simulink model "UrbanCHIL"  (Simulink 8.1)
settings: Solver=ode1  StartTime=0.0  StopTime=inf  FixedStep=Ts  MaxStep=1e-3  RelTol=1e-3
PostLoadFcn:
  | NREL_Mode=1; BANSHEE_init;
InitFcn:
  | NREL_Mode=1; BANSHEE_init;
values from neighbouring files (symbols this model uses):
  DER_REL = xlsread('DER_relay.xlsx')    [relay_settings_init.m]
  F0 = xlsread('F0_relay_banshee.xlsx')    [relay_settings_init.m]
  F2 = xlsread('F2_relay_banshee.xlsx')    [relay_settings_init.m]
  F3 = xlsread('F3_relay_banshee.xlsx')    [relay_settings_init.m]
  F4 = xlsread('F4_relay_nrel.xlsx')    [relay_settings_init.m]
  Ts = 100E-6    (= 0.0001)    [BANSHEE_init.m]    (also in Ghost_init.m)
undefined symbols (not defined in the file or in its folder): CBID, communications_lib, Feeder2_lib, Feeder3_lib, Feeder4_lib, generic_ethernet_cb, Left, relay_housing_lib, SM_UtilityService, SS_COMMUNICATION, SS_F2_RELAY_HOUSING, SS_F3_RELAY_HOUSING, SS_Feeder2, SS_Feeder3, SS_Feeder4, Stim, type, utility_service_lib, V
libraries: simulink x80, relay_modbus_lib x80, breaker_lib x46, rtio_generic_modbus x45, cables_lib x30, rtlab x22, Load_lib x21, powerlib x20, transformer_lib x19, ssn_lib x13, artemis x6, BESS_lib x4
(part 6 of 6)

== system UrbanCHIL/SS_COMMUNICATION/Relay_data/ExtractF3 ==
  In1 : Inport
  Bus Selector47 : BusSelector  OutputSignals=F3_CB_1,F3_CB_2,F3_CB_3,F3_CB_4,F3_CB_5,F3_CB_6,F3_CB_7,F3_CB_8,F3_CB_9,F3_CB_10
  Bus Selector{48..53,56,58..59,61} (10 alike) : BusSelector  OutputSignals=m.kw,m.kvar,m.Vpu,m.Hz,m.status  OutputAsBus=on
  Mux13 : Mux  Inputs=10
  Out1 : Outport
  wires:
  Bus Selector51/1 -> Mux13/5
  Bus Selector48/1 -> Mux13/1
  Bus Selector53/1 -> Mux13/7
  Bus Selector47/4 -> Bus Selector50/1  "<F3_CB_4>"
  Bus Selector47/1 -> Bus Selector48/1  "<F3_CB_1>"
  Bus Selector50/1 -> Mux13/4
  In1/1 -> Bus Selector47/1
  Mux13/1 -> Out1/1
  Bus Selector52/1 -> Mux13/6
  Bus Selector56/1 -> Mux13/8
  Bus Selector58/1 -> Mux13/9
  Bus Selector47/6 -> Bus Selector52/1  "<F3_CB_6>"
  Bus Selector47/7 -> Bus Selector53/1  "<F3_CB_7>"
  Bus Selector47/8 -> Bus Selector56/1  "<F3_CB_8>"
  Bus Selector47/9 -> Bus Selector58/1  "<F3_CB_9>"
  Bus Selector47/3 -> Bus Selector61/1  "<F3_CB_3>"
  Bus Selector47/2 -> Bus Selector49/1  "<F3_CB_2>"
  Bus Selector49/1 -> Mux13/2
  Bus Selector47/10 -> Bus Selector59/1  "<F3_CB_10>"
  Bus Selector47/5 -> Bus Selector51/1  "<F3_CB_5>"
  Bus Selector59/1 -> Mux13/10
  Bus Selector61/1 -> Mux13/3

== system UrbanCHIL/SS_COMMUNICATION/Relay_data/ExtractF4 ==
  In1 : Inport
  Bus Selector47 : BusSelector  OutputSignals=F4_CB_1,F4_CB_2,F4_CB_3,F4_CB_4,F4_CB_5,F4_CB_6
  Bus Selector{48..52,61} (6 alike) : BusSelector  OutputSignals=m.kw,m.kvar,m.Vpu,m.Hz,m.status  OutputAsBus=on
  Mux13 : Mux  Inputs=6
  Out1 : Outport
  wires:
  Bus Selector61/1 -> Mux13/3
  Bus Selector47/5 -> Bus Selector51/1  "<F4_CB_5>"
  Bus Selector49/1 -> Mux13/2
  Bus Selector47/2 -> Bus Selector49/1  "<F4_CB_2>"
  Bus Selector47/3 -> Bus Selector61/1  "<F4_CB_3>"
  Bus Selector47/6 -> Bus Selector52/1  "<F4_CB_6>"
  Bus Selector52/1 -> Mux13/6
  Mux13/1 -> Out1/1
  In1/1 -> Bus Selector47/1
  Bus Selector50/1 -> Mux13/4
  Bus Selector47/1 -> Bus Selector48/1  "<F4_CB_1>"
  Bus Selector47/4 -> Bus Selector50/1  "<F4_CB_4>"
  Bus Selector48/1 -> Mux13/1
  Bus Selector51/1 -> Mux13/5

== system UrbanCHIL/SS_COMMUNICATION/Relay_data/Subsystem ==
  F2 : Inport
  F3 : Inport  Port=2
  Bus Selector1 : BusSelector  OutputSignals=F2_PCC
  Bus Selector2 : BusSelector  OutputSignals=m.kw,m.kvar,m.Vpu,m.Hz,m.status  OutputAsBus=on
  Bus Selector3 : BusSelector  OutputSignals=F3_PCC
  Bus Selector4 : BusSelector  OutputSignals=m.kw,m.kvar,m.Vpu,m.Hz,m.status  OutputAsBus=on
  Constant3 : Constant  Value=zeros(1,5)
  Mux : Mux  Inputs=3
  Out1 : Outport
  wires:
  Constant3/1 -> Mux/1
  Bus Selector1/1 -> Bus Selector2/1  "<F2_PCC>"
  F2/1 -> Bus Selector1/1
  Bus Selector2/1 -> Mux/2
  Bus Selector3/1 -> Bus Selector4/1  "<F3_PCC>"
  F3/1 -> Bus Selector3/1
  Bus Selector4/1 -> Mux/3
  Mux/1 -> Out1/1

== system UrbanCHIL/SS_COMMUNICATION/Relay_data/Subsystem1 ==
  F2 : Inport
  F3 : Inport  Port=2
  F4 : Inport  Port=3
  Bus Selector1 : BusSelector  OutputSignals=ESS_DATA,PV_DATA
  Bus Selector10 : BusSelector  OutputSignals=m.kw,m.kvar,m.Vpu,m.Hz,m.status  OutputAsBus=on
  Bus Selector11 : BusSelector  OutputSignals=cb.relay_out
  Bus Selector{2,6,12,17} (4 alike) : BusSelector  OutputSignals=CB_meas.relay_out.m.kw,CB_meas.relay_out.m.kvar,CB_meas.relay_out.m.Vpu,CB_meas.relay_out.m.Hz,CB_meas.cb_meas.Status  OutputAsBus=on
  Bus Selector16 : BusSelector  OutputSignals=cb.relay_out
  Bus Selector3 : BusSelector  OutputSignals=NG_CHP_DATA
  Bus Selector4 : BusSelector  OutputSignals=m.kw,m.kvar,m.Vpu,m.Hz,m.status  OutputAsBus=on
  Bus Selector9 : BusSelector  OutputSignals=GEN3_DATA,ESS_DATA,PV_DATA
  Constant3 : Constant  Value=zeros(1,5)
  Mux : Mux  Inputs=7
  Out1 : Outport
  wires:
  Mux/1 -> Out1/1
  Bus Selector4/1 -> Mux/4
  F3/1 -> Bus Selector3/1
  Bus Selector3/1 -> Bus Selector16/1  "<NG_CHP_DATA>"
  Bus Selector6/1 -> Mux/2
  F2/1 -> Bus Selector1/1
  Bus Selector1/1 -> Bus Selector6/1  "<ESS_DATA>"
  Constant3/1 -> Mux/1
  Bus Selector1/2 -> Bus Selector2/1  "<PV_DATA>"
  Bus Selector2/1 -> Mux/3
  F4/1 -> Bus Selector9/1
  Bus Selector9/1 -> Bus Selector11/1  "<GEN3_DATA>"
  Bus Selector11/1 -> Bus Selector10/1  "<relay_out>"
  Bus Selector10/1 -> Mux/5
  Bus Selector17/1 -> Mux/6
  Bus Selector9/3 -> Bus Selector12/1  "<PV_DATA>"
  Bus Selector12/1 -> Mux/7
  Bus Selector16/1 -> Bus Selector4/1  "<relay_out>"
  Bus Selector9/2 -> Bus Selector17/1  "<ESS_DATA>"

== system UrbanCHIL/SS_Feeder4/PV2/PV model ==
  note: PV Model
  note: Note Delay was 1
  note: Number of series modules per string
  note: Number of parallel strings in an array
  note: ambient temperature
  note: for 500kW PV rating at 450V:
      | Ns = 30 and Np = 35
  note: for 250kW PV rating at 450V:
      | Ns = 30 and Np = 18
  note: for 550kW PV rating at 450V:
      | Ns = 30 and Np = 39
  note: for 450kW PV rating at 450V:
      | Ns = 30 and Np = 32
  note: for 500kW PV rating at 500V:
      | Ns = 34 and Np = 32
  note: 1 PV module ratings @ 1000 W/m2:
      | Pm = 92.7674 W
      | Vm = 15 V
      | Im = 6.1845 A
  note: for 550kW PV rating at 500V:
      | Ns = 34 and Np = 35
  note: when using only two mangna units:
  note: for 250kW PV rating at 500V:
      | Ns = 34 and Np = 40
  note: when using 5 magna units:
  note: for 250kW PV rating at 450V:
      | Ns = 30 and Np = 45
  note: for 200kW PV rating at 450V:
      | Ns = 30 and Np = 36
  note: for 200kW PV rating at 500V:
      | Ns = 34 and Np = 32
  note: when using only one mangna units:
  note: for 110kW PV rating at 450V:
      | Ns = 30 and Np = 39
  note: for 100kW PV rating at 450V:
      | Ns = 30 and Np = 36
  note: for 100kW PV rating at 500V:
      | Ns = 34 and Np = 32
  note: for 110kW PV rating at 500V:
      | Ns = 34 and Np = 35
  Vdc_meas : Inport
  Idc_meas : Inport  Port=2
  Tamb : Inport  Port=3
  POA_Insolation : Inport  Port=4
  SeriesN : Inport  Port=5
  ParallelN : Inport  Port=6
  Imin : Inport  Port=7
  " 3" : Terminator
  -60 to +80 C : Saturate  UpperLimit=80  LowerLimit=-60
  0 to 1500 W/m^2 : Saturate  UpperLimit=1500  LowerLimit=0
  1 to 600 V : Saturate  UpperLimit=600  LowerLimit=1
  First-Order Filter : powerlib_meascontrol/Filters/First-Order Filter  FilterType=Lowpass  Tc=200e-3  Ts=100e-6  Initialize=on  Vac_Init=[0, 0, 60]  Vdc_Init=0  PlotResponse=off  FreqRange="[0,  200,  1]"
  First-Order Filter1 : powerlib_meascontrol/Filters/First-Order Filter  FilterType=Lowpass  Tc=200e-3  Ts=100e-6  Initialize=on  Vac_Init=[0, 0, 60]  Vdc_Init=0  PlotResponse=off  FreqRange="[0,  200,  1]"
  Imin1 : Constant  Value=0
  MATLAB Function : MATLAB Function  TreatAsAtomicUnit=on
  Saturation Dynamic : simulink/Discontinuities/Saturation Dynamic  OutMin=[]  OutMax=[]  OutDataTypeStr=Inherit: Same as second input  OutDataType=fixdt(1, 16)  OutScaling=2^-10  DoSatur=off
  Vpv_set : Outport
  Ipv_set : Outport  Port=2
  wires:
  Imin1/1 -> MATLAB Function/7(Iout_old)
  SeriesN/1 -> MATLAB Function/1(Ns_module)
  ParallelN/1 -> MATLAB Function/2(Np_string)
  Tamb/1 -> -60 to +80 C/1
  POA_Insolation/1 -> 0 to 1500 W/m^2/1
  Vdc_meas/1 -> First-Order Filter/1
  Saturation Dynamic/1 -> Ipv_set/1
  0 to 1500 W/m^2/1 -> MATLAB Function/5(G)
  -60 to +80 C/1 -> MATLAB Function/4(Tamb)
  1 to 600 V/1 -> MATLAB Function/3(Vin)
  Idc_meas/1 -> First-Order Filter1/1
  First-Order Filter/1 -> 1 to 600 V/1
  First-Order Filter1/1 -> MATLAB Function/6(Imeas)
  MATLAB Function/4(Iout) -> Saturation Dynamic/2  "Iout"
  Imin/1 -> Saturation Dynamic/3
  MATLAB Function/3(IscMax) -> Saturation Dynamic/1  "IscMax"
  MATLAB Function/2(VocMax) -> " 3"/1  "VocMax"
  MATLAB Function/1(Vout) -> Vpv_set/1  "Vout"

== system UrbanCHIL/SS_COMMUNICATION/NREL UDP Data - Formatted Packets/Number of seconds of recording/Increment ==
  Trigger : TriggerPort
  Increment : Constant
  Memory : Memory  InheritSampleTime=on
  Sum : Sum  Inputs=|++
  Out1 : Outport
  wires:
  Sum/1 -> Out1/1, Memory/1
  Memory/1 -> Sum/1
  Increment/1 -> Sum/2

== matlab function SS_Feeder4/PV2/PV model/MATLAB Function ==
  data: Ns_module input double; Vout output double; VocMax output double; IscMax output double; Np_string input double; Vin input double; Tamb input double; G input double; Imeas input double; Iout_old input double; Iout output double
function [Vout, VocMax, IscMax, Iout]  = bp_sx110(Ns_module, Np_string, Vin, Tamb, G, Imeas, Iout_old)
%
% function bp_sx110.m models the BP SX 110 PV module
%	module date found at: http://www.posharp.com/bp-sx110-solar-panel-from-bp-solar_p60866579d.aspx
%
% P.S.: according to: https://www.homepower.com/view/?file=HP113_pg106_WordPower
%	PV array ---> set of parallel and series modules
%	PV module (sometimes called panel) ---> set of parallel and series PV cells
%	PV string ---> set of series connected modules (panels)
%
% The function calculates array output current under given:
%	1- number of modules in series (modules in a string)
%	2- number of strings in parallel
%	3- irradiance and temperature
%
% This model was written by Noel Dillman and Blake Lundstrom of the Colorado School of Mines while working on a project for the National
% 	Renewable Energy Laboratory.
% It was further improved by Ali Hariri (research intern from CAPS-FSU) on June 6th, 2016. The code is made more consistent interms of
% 	terminology; more comments were added with references for better use in future work.
% It is based on the original bp_sx110 model created by Akihiro Oi (California Polytechnic State University) on 07/01/2005 
%	(see "Design and Simulation of Photovoltaic Water Pumping System" (September 2005)).
% Further PV model modifications were made based on the model presented in "Comprehensive Approach to Modeling and Simulation of 
% 	Photovoltaic Arrays" (2009) by Villalva et al.
% 
% Out:  Vout = array output voltage
%       Iout = Output current
%       VocMax = Open-Circuit Voltage
%       IscMax = Short-Circuit Current
% In:   Ns_module = Number of modules in series per string
%       Np_string = Number of strings in parallel
%       Tamb = ambient temperature in degrees celsius
%       G = Irradiance (1G = 1000 W/m^2) (can be input in W/m^2 or kW/m^2)
%       Vin = Voltage of load
%       Iout_old = Feedback loop from previous Iout

% *************************************************************************
%   Start Code
% *************************************************************************
Imeas = Imeas / 2;  % since we are using 5 modules of the magna power
                    % this code calculates the output for 1 

% if G is given in 1 W/m^2, convert to 1000 W/m^2
if G > 1.5
    G = G / 1000;
end

% Set all negative irradiances to 0
if G < 0
    G = 0;
end

% *************************************************************************
%   determine cell temperature from irradiance, windspeed, ambient temperature, and SAPM (sandia array performance model) module parameters
%		using King's SFP model (see pvl_sapmcelltemp): https://pvpmc.sandia.gov/PVLIB_Matlab_Help/html/pvl_sapmcelltemp_help.html
% *************************************************************************
G0 = 1000;                                          % reference irradiance type 1000 W/m2
windspeed = 10;                                     % use a default value for windspeed since its a second order effect
ap = -3.47;                                         % default for SAM glass/cell/glass
b = -0.0594;        %
deltaT = 3;         %
Tmodule = Tamb + (G*1000)*(exp(ap + b*windspeed));  % module temperature in degrees
Tcell_C = Tmodule + (G*1000/G0)*deltaT;				% cell temperature in degrees
Tcell_K = 273 + Tcell_C;                            % cell temperature in Kelvin

% *************************************************************************
%   Define and Calculate Constants and Variables
% *************************************************************************
% PV cell data
% ---------------------------------------------------------------------------------------
derating = 0.921;                                   % Panel derating factor
k = 1.381e-23;                                      % Boltzmanns constant
q = 1.602e-19;                                      % Electron charge
a = 1.25;                                           % Diode ideality factor (n),1 (ideal diode) < n < 2
Res = 400;                                          % I-V curve resolution - adjustable
Rs = 0.001;                                         % Series resistance per cell
Rp = 2;                                             % Parallel resistance per cell
TrK = 298;                                          % Reference temperature (25C) in Kelvin
Kv = -0.08;                                         % Voltage temperature coefficient (-80mV/C)
Ki = 0.65e-3;                                       % Temperature coefficient of Isc (0.065%/C)
% ---------------------------------------------------------------------------------------

% calculate module data
% ---------------------------------------------------------------------------------------
Ns_cell = 36*Ns_module;                               		% total number of series connected cells (BP SX110, 36 series cells per module)
Voc_TrK_module = 20.1;                                		% Voc in volts per module @ reference temp (V/panel)
Voc_TaK_module = Voc_TrK_module + (Kv*(Tcell_K - TrK));     % Voc per module @ actual temp
Voc = Voc_TaK_module/36;                              		% Voc per cell @ actual temp
Isc_nameplate = 7.38;                                 		% Isc per cell given on nameplate
Isc_TrK = Isc_nameplate*derating;                     		% Isc (short circuit current per cell) @ reference temp inclusive of derating
% ---------------------------------------------------------------------------------------

% *************************************************************************
%   Calculate outputs
% *************************************************************************

Isc = G *(Isc_TrK * (1 + (Ki * (Tcell_K - TrK))));      % Calculate PV cell short-circuit 'I' for given temp and irradiance
Vt =  k * Tcell_K / q;                                  % Define PV cell thermal potential (Vt) at actual temp
VocMax  = Voc_TaK_module*Ns_module;                     % max Voc per array due to temperature

% Set Vin to VocMax if requested Vin is beyond scope
if Vin > VocMax
    Vin = VocMax;
end
% ---------------------------------------------------------------------------------------

% If Vin is small, it is either startup or Isc.
% If it is Isc then Iout_old should be nearly Isc
if Vin < 1
    iTol = abs(Isc - (Iout_old/Np_string)) / (Iout_old/Np_string);
    % if Iout_old is within 5% of Isc
    if(iTol < 0.05)
        %use normal Vin value
    else
        %set Vout = Vin = Voc
        Vin = Ns_cell*Voc;
    end
end
% ---------------------------------------------------------------------------------------

Vc = Vin / Ns_cell;                                     	% Range of individual cell voltages of array
Io = Isc / (exp(Voc /(a* Vt)) -1);							% reverse saturation current for given temperature per cell
Id = (Io*(exp((Vc + (Iout_old/Np_string)*Rs)/(a*Vt))-1));  	% Diode + Series Resistance Current
Ip = (Vc + (Iout_old/Np_string)*Rs)/Rp;                    	% Parallel Resistance Current
Ia = Isc - Id - Ip;                            	% Final PV current (cell output)
% ---------------------------------------------------------------------------------------

% capture any negative commands to Ia out before they leave the block.
% This avoids negatives in the Ia delay feedback
% Ia1 = Np_string*Ia; % array output
if Ia < 0 
    Ia = 0;
end

IscMax = Isc*Np_string;
Vout = Vin;
% If Imeas is small (<10% of Isc) assume that we are at startup and set Iout = IscMax*0.3 
% (0.3 is chosen arbitrary smaller than Iscmax) otherwise use Ia
% if (Imeas <= 0.1 * IscMax)
%     Iout = IscMax * 0.3;
% else
%     Iout = Np_string*Ia;
% end
Iout = Np_string*Ia;

== matlab function SS_COMMUNICATION/NREL UDP Data - Formatted Packets/Cast uint16 ==
  data: u input double; y output double
function y = fcn(u)
%#codegen

x = double(typecast(uint32(u),'uint16'));
y = x(1); % low bits
